simulink model "untitled"  (R2024b)
settings: Solver=VariableStepAuto  StartTime=0.0  StopTime=10.0  MaxStep=0.001  RelTol=1e-3
libraries: simulink x1
settings Model: Creator=Administrator  LastModifiedBy=Administrator

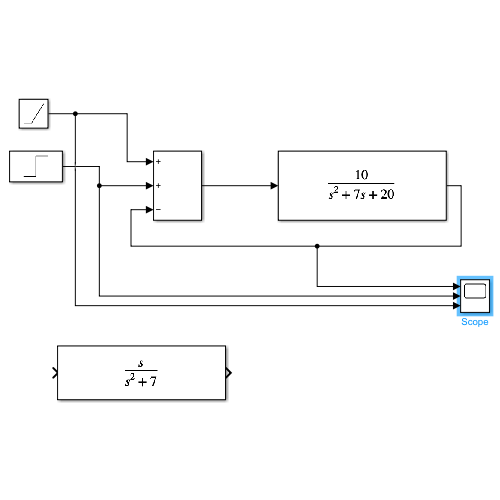
[thumbnail: Simulink's stored preview of the top-level diagram]
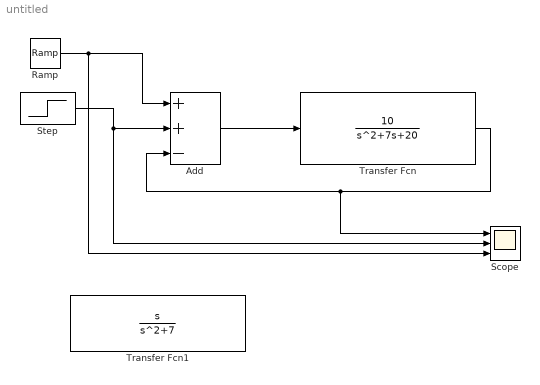
== system untitled ==
  Add : Sum  Inputs=++-
  Ramp : simulink/Sources/Ramp  slope=0.1  start=3  InitialOutput=0
  Scope : Scope  NumInputPorts=3
  Step : Step  SampleTime=0
  Transfer Fcn : TransferFcn  Numerator=[10]  Denominator=[1 7 20]
  Transfer Fcn1 : TransferFcn  Numerator=[0 1 0]  Denominator=[1 0 7]
  wires:
  Step/1 -> Scope/2, Add/2
  Add/1 -> Transfer Fcn/1
  Transfer Fcn/1 -> Scope/1, Add/3
  Ramp/1 -> Scope/3, Add/1
